simulink library "models"  (Simulink 7.2)
settings: Solver=ode45  SolverMode=SingleTasking  StartTime=0.0  StopTime=10.0  RelTol=1e-3
undefined symbols (not defined in the file or in its folder): actuator_T2_lib, aero, Aero, aero_lib, aftfuel, aftfuel_pos, Am, atmos, b, bias, Bm, Cbar, cg_pos0, cg_shift_gear, constants, DamageModels, Ed_trim_IC, engl_ang, engl_pos, engr_ang, engr_pos, fwdfuel, fwdfuel_pos, GTM_T2, hd_trim_IC, in_tadapton_forced, Inertia0, Inertia_shift_gear, latlonh_IC, MACH_U_nom_IC, Nd_trim_IC, pqr_trim_IC, quat_trim_IC, ref_cg, S, SENSOR, SERVO, symmetric_aero_on, trac_params, use_wind_meas_sim, vehicle_params, w0, xm0
libraries: simulink_need_slupdate x56, models x11, aeroutilslib x6, utility_lib x5, GTM_aerolib x4, model_lib x4, Polyval_lib x3, simulink x2, enginelib x2, engine_T2_lib x1
(part 2 of 4)

== system models/gtm-aero (for V0905)/AuxVars_Reduced ==
  pqr : Inport  OutDataType=sfix(16)  OutScaling=2^0
  aero_env : Inport  Port=2  OutDataType=sfix(16)  OutScaling=2^0
  P : Inport  Port=3  OutDataType=sfix(16)  OutScaling=2^0
  T : Inport  Port=4  OutDataType=sfix(16)  OutScaling=2^0
  Bus Creator : BusCreator  Inputs=6
  Bus Creator1 : BusCreator  Inputs=3
  Bus Selector : BusSelector  OutputSignals=qbar,alpha,beta,vel
  Demux : Demux  Outputs=3
  Gain : Gain  Gain=1/atmos.alt_T0  ParameterDataType=sfix(16)  ParameterScaling=2^0  OutDataType=sfix(16)  OutScaling=2^0
  Gain1 : Gain  Gain=1/atmos.alt_P0  ParameterDataType=sfix(16)  ParameterScaling=2^0  OutDataType=sfix(16)  OutScaling=2^0
  Gain2 : Gain  Gain=180/pi  ParameterDataType=sfix(16)  ParameterScaling=2^0  OutDataType=sfix(16)  OutScaling=2^0
  Gain3 : Gain  Gain=180/pi  ParameterDataType=sfix(16)  ParameterScaling=2^0  OutDataType=sfix(16)  OutScaling=2^0
  Gain5 : Gain  Gain=1/1.689  ParameterDataType=sfix(16)  ParameterScaling=2^0  OutDataType=sfix(16)  OutScaling=2^0
  AuxVars : Outport  OutDataType=sfix(16)  OutScaling=2^0
  State : Outport  Port=2  OutDataType=sfix(16)  OutScaling=2^0
  wires:
  Gain3/1 -> Bus Creator/3  "beta"
  Gain2/1 -> Bus Creator/2  "alpha"
  aero_env/1 -> Bus Selector/1
  P/1 -> Gain1/1
  T/1 -> Gain/1
  Gain1/1 -> Bus Creator/5  "pratio"
  pqr/1 -> Demux/1
  Demux/1 -> Bus Creator1/1  "pb"
  Demux/2 -> Bus Creator1/2  "qb"
  Demux/3 -> Bus Creator1/3  "rb"
  Bus Creator1/1 -> State/1
  Bus Selector/1 -> Bus Creator/1  "<qbar>"
  Bus Selector/2 -> Gain2/1  "<alpha>"
  Bus Selector/3 -> Gain3/1  "<beta>"
  Bus Selector/4 -> Gain5/1  "<vel>"
  Gain/1 -> Bus Creator/6  "tratio"
  Bus Creator/1 -> AuxVars/1
  Gain5/1 -> Bus Creator/4  "tas"

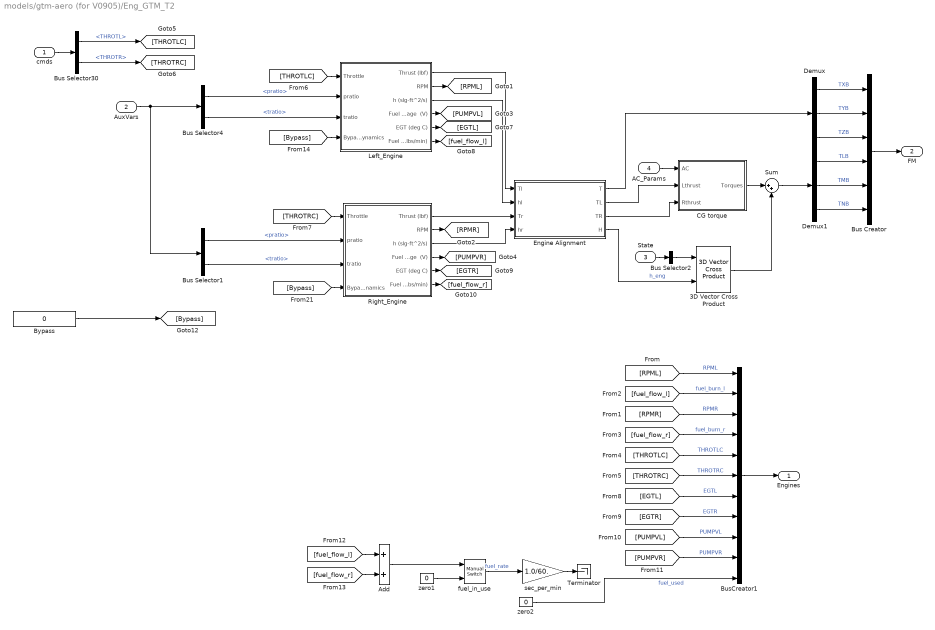
== system models/gtm-aero (for V0905)/Eng_GTM_T2 ==
  cmds : Inport  OutDataType=sfix(16)  OutScaling=2^0
  AuxVars : Inport  Port=2  OutDataType=sfix(16)  OutScaling=2^0
  State : Inport  Port=3  OutDataType=sfix(16)  OutScaling=2^0
  AC_Params : Inport  Port=4  OutDataType=sfix(16)  OutScaling=2^0
  3D Vector Cross Product : aeroutilslib/3D Vector Cross Product  SystemSampleTime=-1
  Add : Sum  OutDataType=sfix(16)  OutScaling=2^-10
  Bus Creator : BusCreator  Inputs=6
  Bus Selector1 : BusSelector  OutputSignals=pratio,tratio
  Bus Selector2 : BusSelector  OutputSignals=pb,qb,rb  OutputAsBus=on
  Bus Selector30 : BusSelector  OutputSignals=THROTL,THROTR
  Bus Selector4 : BusSelector  OutputSignals=pratio,tratio
  BusCreator1 : BusCreator  Inputs=11
  Bypass : Constant  Value=0  OutDataType=sfix(16)  OutScaling=2^0
  CG torque : Subsystem
  Demux : Demux  Outputs=3
  Demux1 : Demux  Outputs=3
  Engine Alignment : Stateflow chart
  Left_Engine : Subsystem  BlockChoice=Jetcat P70b
      settings: AttributesFormatString=%<BlockChoice>  TemplateBlock=enginelib/Engine Model  MemberBlocks=AMT-180,AMT-280,Blank,Jetcat P120SE,Jetcat P70,Jetcat P70b
  Right_Engine : Subsystem  BlockChoice=Jetcat P70b
      settings: AttributesFormatString=%<BlockChoice>  TemplateBlock=enginelib/Engine Model  MemberBlocks=AMT-180,AMT-280,Blank,Jetcat P120SE,Jetcat P70,Jetcat P70b
  Sum : Sum  Inputs=|++  OutDataType=sfix(16)  OutScaling=2^0
  Terminator : Terminator
  fuel_in_use : simulink/Signal Routing/Manual Switch  SystemSampleTime=-1  sw=0  action=0  varsize=off
  sec_per_min : Gain  Gain=1.0/60.  ParameterDataType=sfix(16)  ParameterScaling=2^0  OutDataType=sfix(16)  OutScaling=2^0  SaturateOnIntegerOverflow=on  OutDataTypeStr=Inherit: Same as input  ParamDataTypeStr=Inherit: Same as input
  zero1 : Constant  Value=0  OutDataType=sfix(16)  OutScaling=2^0
  zero2 : Constant  Value=0  OutDataType=sfix(16)  OutScaling=2^0
  Engines : Outport  OutDataType=sfix(16)  OutScaling=2^0
  FM : Outport  Port=2  PortDimensions=6  OutDataType=sfix(16)  OutScaling=2^0
  wires:
  Right_Engine/6(Fuel Flow (lbs/min)) -> [fuel_flow_r]
  Right_Engine/5(EGT (deg C)) -> [EGTR]
  Left_Engine/6(Fuel Flow (lbs/min)) -> [fuel_flow_l]
  Left_Engine/5(EGT (deg C)) -> [EGTL]
  cmds/1 -> Bus Selector30/1
  Demux/2 -> Bus Creator/2  "TYB"
  State/1 -> Bus Selector2/1
  Bus Selector2/1 -> 3D Vector Cross Product/1
  Demux/3 -> Bus Creator/3  "TZB"
  Left_Engine/2(RPM) -> [RPML]
  Left_Engine/4(Fuel Pump Voltage  (V)) -> [PUMPVL]
  Right_Engine/4(Fuel Pump Voltage  (V)) -> [PUMPVR]
  Right_Engine/2(RPM) -> [RPMR]
  Bus Selector1/1 -> Right_Engine/2(pratio)  "<pratio>"
  Bus Selector1/2 -> Right_Engine/3(tratio)  "<tratio>"
  AuxVars/1 -> Bus Selector1/1, Bus Selector4/1
  AC_Params/1 -> CG torque/1(AC)
  Bus Creator/1 -> FM/1
  Bus Selector30/1 -> [THROTLC]  "<THROTL>"
  Bus Selector30/2 -> [THROTRC]  "<THROTR>"
  [THROTLC] -> Left_Engine/1(Throttle)
  [THROTRC] -> Right_Engine/1(Throttle)
  [THROTRC] -> BusCreator1/6  "THROTRC"
  [THROTLC] -> BusCreator1/5  "THROTLC"
  [fuel_flow_r] -> BusCreator1/4  "fuel_burn_r"
  [fuel_flow_l] -> BusCreator1/2  "fuel_burn_l"
  [RPMR] -> BusCreator1/3  "RPMR"
  [RPML] -> BusCreator1/1  "RPML"
  BusCreator1/1 -> Engines/1
  [EGTL] -> BusCreator1/7  "EGTL"
  [EGTR] -> BusCreator1/8  "EGTR"
  [PUMPVL] -> BusCreator1/9  "PUMPVL"
  [PUMPVR] -> BusCreator1/10  "PUMPVR"
  sec_per_min/1 -> Terminator/1
  fuel_in_use/1 -> sec_per_min/1  "fuel_rate"
  zero2/1 -> BusCreator1/11  "fuel_used"
  [fuel_flow_l] -> Add/1
  [fuel_flow_r] -> Add/2
  zero1/1 -> fuel_in_use/2
  Add/1 -> fuel_in_use/1
  Bus Selector4/1 -> Left_Engine/2(pratio)  "<pratio>"
  Bus Selector4/2 -> Left_Engine/3(tratio)  "<tratio>"
  [Bypass] -> Left_Engine/4(BypassDynamics)
  [Bypass] -> Right_Engine/4(BypassDynamics)
  Bypass/1 -> [Bypass]
  Left_Engine/1(Thrust (lbf)) -> Engine Alignment/1(Tl)
  Right_Engine/1(Thrust (lbf)) -> Engine Alignment/3(Tr)
  Demux/1 -> Bus Creator/1  "TXB"
  Left_Engine/3(h (slg-ft^2/s)) -> Engine Alignment/2(hl)
  Right_Engine/3(h (slg-ft^2/s)) -> Engine Alignment/4(hr)
  Engine Alignment/4(H) -> 3D Vector Cross Product/2  "h_eng"
  Engine Alignment/1(T) -> Demux/1
  Engine Alignment/2(TL) -> CG torque/2(Lthrust)
  Engine Alignment/3(TR) -> CG torque/3(Rthrust)
  CG torque/1(Torques) -> Sum/1
  3D Vector Cross Product/1 -> Sum/2
  Sum/1 -> Demux1/1
  Demux1/1 -> Bus Creator/4  "TLB"
  Demux1/2 -> Bus Creator/5  "TMB"
  Demux1/3 -> Bus Creator/6  "TNB"

== system models/gtm-aero (for V0905)/aero surf ganging ==
  u : Inport  OutDataType=sfix(16)  OutScaling=2^0
  Actuator_GTM_T2 (modified) : Subsystem  AncestorBlock=actuator_T2_lib/GTM_T2
  Input Generator (modified) : Subsystem  AncestorBlock=UserContent_lib/Input Generator
  cmds : Outport  OutDataType=sfix(16)  OutScaling=2^0
  wires:
  Input Generator (modified)/2(cmd_stab) -> Actuator_GTM_T2 (modified)/2(cmd_stab)
  Actuator_GTM_T2 (modified)/1(Surface Pos) -> cmds/1
  Input Generator (modified)/1(cmds) -> Actuator_GTM_T2 (modified)/1(cmds)
  u/1 -> Input Generator (modified)/1(Feedback)

== system models/tmp - 1st order sensor model/1st order sensor model ==
  note: VARIABLE RATE LIMIT SERVO MODEL
      | (1st order)
  act_bus : Inport  OutDataType=sfix(16)  OutScaling=2^0
  Bus Selector1 : BusSelector  OutputSignals=effector_limits.u_ulim,effector_limits.u_llim,effector_limits.u_urlim,effector_limits.u_lrlim,u_cmd
  Enforce lower limit : MinMax  Function=max  Inputs=2  OutDataType=sfix(16)  OutScaling=2^-10  OutDataTypeStr=Inherit: Inherit via back propagation  ZeroCross=off
  Enforce lower limit1 : MinMax  Function=max  Inputs=2  OutDataType=sfix(16)  OutScaling=2^-10  OutDataTypeStr=Inherit: Inherit via back propagation  ZeroCross=off
  Enforce upper limit : MinMax  Inputs=2  OutDataType=sfix(16)  OutScaling=2^-10  OutDataTypeStr=Inherit: Inherit via back propagation  ZeroCross=off
  Enforce upper limit1 : MinMax  Inputs=2  OutDataType=sfix(16)  OutScaling=2^-10  OutDataTypeStr=Inherit: Inherit via back propagation  ZeroCross=off
  Sum : Sum  Inputs=|+-  OutDataType=sfix(16)  OutScaling=2^0  SaturateOnIntegerOverflow=on  InputSameDT=on  OutDataTypeStr=Inherit: Same as first input
  Sum1 : Sum  Inputs=|++  OutDataType=sfix(16)  OutScaling=2^0  SaturateOnIntegerOverflow=on  InputSameDT=on  OutDataTypeStr=Inherit: Same as first input
  Sum2 : Sum  Orientation=left  Inputs=-+|  OutDataType=sfix(16)  OutScaling=2^0  SaturateOnIntegerOverflow=on  InputSameDT=on  OutDataTypeStr=Inherit: Same as first input
  W : Gain  Gain=SERVO.w  ParameterDataType=sfix(16)  ParameterScaling=2^0  OutDataType=sfix(16)  OutScaling=2^0  SaturateOnIntegerOverflow=on  OutDataTypeStr=Inherit: Same as input  ParamDataTypeStr=Inherit: Same as input
  anti-windup gain : Gain  Orientation=left  Gain=SERVO.pos_Kaw  ParameterDataType=sfix(16)  ParameterScaling=2^0  OutDataType=sfix(16)  OutScaling=2^0
  pos integrator : Integrator  InitialCondition=SERVO.x0
  u_pos : Outport  OutDataType=sfix(16)  OutScaling=2^0
  wires:
  Enforce upper limit1/1 -> Sum1/1
  Enforce lower limit1/1 -> Enforce upper limit1/2
  W/1 -> Enforce lower limit1/2
  Bus Selector1/3 -> Enforce upper limit1/1  "<u_urlim>"
  Bus Selector1/2 -> Enforce lower limit/1  "<u_llim>"
  Bus Selector1/5 -> Sum/1  "<u_cmd>"
  Sum/1 -> W/1
  Sum1/1 -> pos integrator/1
  anti-windup gain/1 -> Sum1/2
  Sum2/1 -> anti-windup gain/1
  pos integrator/1 -> Enforce lower limit/2, Sum2/1
  Enforce lower limit/1 -> Enforce upper limit/2
  Enforce upper limit/1 -> u_pos/1, Sum/2, Sum2/2
  act_bus/1 -> Bus Selector1/1
  Bus Selector1/1 -> Enforce upper limit/1  "<u_ulim>"
  Bus Selector1/4 -> Enforce lower limit1/1  "<u_lrlim>"

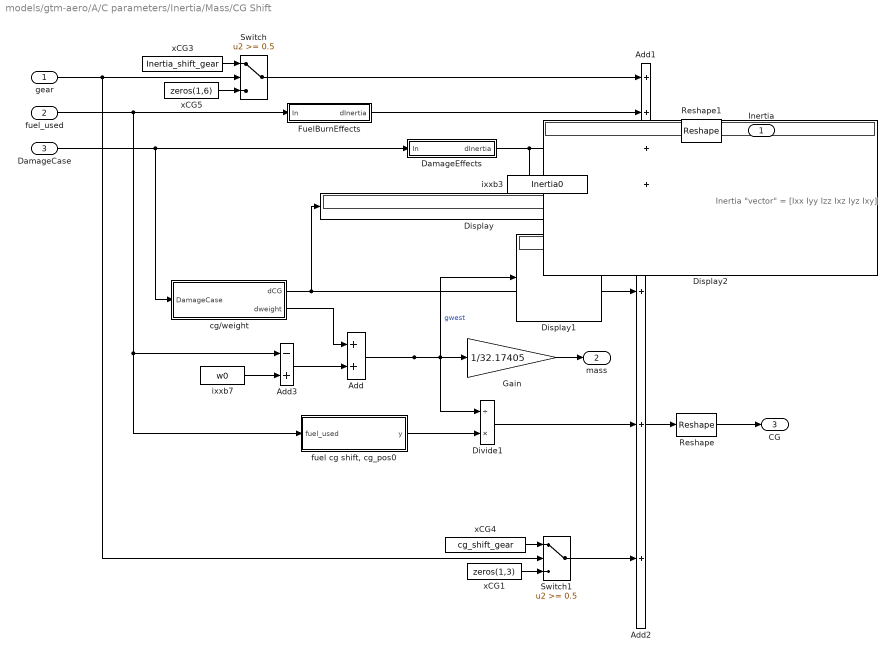
== system models/gtm-aero/A/C parameters/Inertia/Mass/CG Shift ==
  note: Inertia "vector" = [Ixx Iyy Izz Ixz Iyz Ixy]
  gear : Inport  OutDataType=sfix(16)  OutScaling=2^0
  fuel_used : Inport  Port=2  OutDataType=sfix(16)  OutScaling=2^0
  DamageCase : Inport  Port=3  OutDataType=sfix(16)  OutScaling=2^0
  Add : Sum  OutDataType=sfix(16)  OutScaling=2^-10
  Add1 : Sum  Inputs=++++  OutDataType=sfix(16)  OutScaling=2^-10
  Add2 : Sum  Inputs=+++  OutDataType=sfix(16)  OutScaling=2^-10
  Add3 : Sum  Inputs=-+  OutDataType=sfix(16)  OutScaling=2^-10
  DamageEffects : Subsystem
  Display : Display
  Display1 : Display
  Display2 : Display
  Divide1 : Product  Inputs=/*  OutDataType=sfix(16)  OutScaling=2^-10
  FuelBurnEffects : Subsystem
  Gain : Gain  Gain=1/32.17405  ParameterDataType=sfix(16)  ParameterScaling=2^0  OutDataType=sfix(16)  OutScaling=2^0
  Reshape : Reshape
  Reshape1 : Reshape
  Switch : Switch  Threshold=0.5
  Switch1 : Switch  Threshold=0.5
  cg/weight : Subsystem
  "fuel cg shift, cg_pos0" : Stateflow chart
  ixxb3 : Constant  Value=Inertia0  OutDataType=sfix(16)  OutScaling=2^0
  ixxb7 : Constant  Value=w0  OutDataType=sfix(16)  OutScaling=2^0
  xCG1 : Constant  Value=zeros(1,3)  OutDataType=sfix(16)  OutScaling=2^0
  xCG3 : Constant  Value=Inertia_shift_gear  OutDataType=sfix(16)  OutScaling=2^0
  xCG4 : Constant  Value=cg_shift_gear  OutDataType=sfix(16)  OutScaling=2^0
  xCG5 : Constant  Value=zeros(1,6)  OutDataType=sfix(16)  OutScaling=2^0
  Inertia : Outport  OutDataType=sfix(16)  OutScaling=2^0
  mass : Outport  Port=2  OutDataType=sfix(16)  OutScaling=2^0
  CG : Outport  Port=3  OutDataType=sfix(16)  OutScaling=2^0
  wires:
  "fuel cg shift, cg_pos0"/1(y) -> Divide1/2
  Divide1/1 -> Add2/2
  Reshape1/1 -> Inertia/1
  Reshape/1 -> CG/1
  cg/weight/2(dweight) -> Add/1
  gear/1 -> Switch1/2, Switch/2
  cg/weight/1(dCG) -> Display/1, Add2/1
  Add3/1 -> Add/2
  xCG1/1 -> Switch1/3
  xCG4/1 -> Switch1/1
  Switch1/1 -> Add2/3
  ixxb7/1 -> Add3/2
  Gain/1 -> mass/1
  Add2/1 -> Reshape/1
  Add/1 -> Display1/1, Divide1/1, Gain/1  "gwest"
  DamageCase/1 -> cg/weight/1(DamageCase), DamageEffects/1(In)
  DamageEffects/1(dInertia) -> Display2/1, Add1/3
  ixxb3/1 -> Add1/4
  fuel_used/1 -> "fuel cg shift, cg_pos0"/1(fuel_used), Add3/1, FuelBurnEffects/1(In)
  xCG5/1 -> Switch/3
  xCG3/1 -> Switch/1
  Add1/1 -> Reshape1/1
  Switch/1 -> Add1/1
  FuelBurnEffects/1(dInertia) -> Add1/2

== system models/gtm-aero/A/C parameters/TriggerDamage ==
  From Workspace : FromWorkspace  VariableName=[0 0; DamageOnsetTime DamageCase]  Interpolate=off  OutputAfterFinalValue=Holding final value
  damagecase : Outport  OutDataType=sfix(16)  OutScaling=2^0
  wires:
  From Workspace/1 -> damagecase/1

== system models/gtm-aero/Aero_GTM_T2/Coefficent Evaluation ==
  C6 Body : Inport  OutDataType=sfix(16)  OutScaling=2^0
  qbar : Inport  Port=2  OutDataType=sfix(16)  OutScaling=2^0
  Cg : Inport  Port=3  OutDataType=sfix(16)  OutScaling=2^0
  Cp : Inport  Port=4  OutDataType=sfix(16)  OutScaling=2^0
  3D Vector Cross Product : Subsystem  AncestorBlock=aeroutilslib/3D Vector Cross Product
  Demux : Demux  Outputs=[3 3]
  Gain2 : Gain  Gain=Sref  ParameterDataType=sfix(16)  ParameterScaling=2^0  OutDataType=sfix(16)  OutScaling=2^0  SaturateOnIntegerOverflow=on  OutDataTypeStr=Inherit: Same as input  ParamDataTypeStr=Inherit: Same as input
  Product : Product  OutDataType=sfix(16)  OutScaling=2^0  SaturateOnIntegerOverflow=on  InputSameDT=on  OutDataTypeStr=Inherit: Same as first input
  Reference Lengths : Gain  Gain=[b cbar b]  ParameterDataType=sfix(16)  ParameterScaling=2^0  OutDataType=sfix(16)  OutScaling=2^0  SaturateOnIntegerOverflow=on  OutDataTypeStr=Inherit: Same as input  ParamDataTypeStr=Inherit: Same as input
  Sum : Sum  Inputs=-+  OutDataType=sfix(16)  OutScaling=2^0  SaturateOnIntegerOverflow=on
  Sum1 : Sum  Inputs=++|  OutDataType=sfix(16)  OutScaling=2^0  SaturateOnIntegerOverflow=on
  Forces : Outport  OutDataType=sfix(16)  OutScaling=2^0
  Moments : Outport  Port=2  OutDataType=sfix(16)  OutScaling=2^0
  wires:
  Sum/1 -> 3D Vector Cross Product/1(A)
  Cg/1 -> Sum/1
  Cp/1 -> Sum/2
  C6 Body/1 -> Product/1
  qbar/1 -> Product/2
  Product/1 -> Gain2/1
  Gain2/1 -> Demux/1
  Demux/2 -> Reference Lengths/1
  Demux/1 -> 3D Vector Cross Product/2(B), Forces/1
  Reference Lengths/1 -> Sum1/2
  Sum1/1 -> Moments/1
  3D Vector Cross Product/1(AxB) -> Sum1/1

== system models/gtm-aero/Aero_GTM_T2/Dynamic Derviatives ==
  alpha : Inport  OutDataType=sfix(16)  OutScaling=2^0
  beta : Inport  Port=2  OutDataType=sfix(16)  OutScaling=2^0
  TAS : Inport  Port=3  OutDataType=sfix(16)  OutScaling=2^0
  pqr : Inport  Port=4  OutDataType=sfix(16)  OutScaling=2^0
  AC_Params : Inport  Port=5  OutDataType=sfix(16)  OutScaling=2^0
  AC_Params1 : InportShadow  Port=5  OutDataType=sfix(16)  OutScaling=2^0  LatchByCopyingInsideSignal=off
  AC_Params_Dup1 : InportShadow  Port=5  OutDataType=sfix(16)  OutScaling=2^0  LatchByCopyingInsideSignal=off
  Bus Selector : BusSelector  OutputSignals=DamageCase
  Data Type Conversion : DataTypeConversion  OutDataTypeMode=uint32  OutDataType=sfix(16)  OutScaling=2^0  OutDataTypeStr=uint32  RndMeth=Nearest
  Forced Oscillation with Damage Increments : Subsystem
  Merge : Merge  InitialOutput=zeros(6,1)
  Rotary Blended  UnDamaged Case : Subsystem
  Switch Case : SwitchCase  CaseConditions={[1,2,3,4,5,6]}
  TAS1 : InportShadow  Port=3  OutDataType=sfix(16)  OutScaling=2^0  LatchByCopyingInsideSignal=off
  alpha_Dup1 : InportShadow  Port=1  OutDataType=sfix(16)  OutScaling=2^0  LatchByCopyingInsideSignal=off
  pqr_Dup1 : InportShadow  Port=4  OutDataType=sfix(16)  OutScaling=2^0  LatchByCopyingInsideSignal=off
  dC6 : Outport  OutDataType=sfix(16)  OutScaling=2^0
  wires:
  Forced Oscillation with Damage Increments/1(dC6) -> Merge/1
  [ndx] -> Forced Oscillation with Damage Increments/5(DamageCase)
  AC_Params1/1 -> Forced Oscillation with Damage Increments/4(AC_Params)
  pqr_Dup1/1 -> Forced Oscillation with Damage Increments/3(pqr)
  TAS1/1 -> Forced Oscillation with Damage Increments/2(TAS)
  alpha_Dup1/1 -> Forced Oscillation with Damage Increments/1(alpha)
  [ndx] -> Switch Case/1
  Data Type Conversion/1 -> [ndx]
  AC_Params_Dup1/1 -> Bus Selector/1
  Bus Selector/1 -> Data Type Conversion/1  "<DamageCase>"
  Rotary Blended  UnDamaged Case/1(dC6) -> Merge/2
  Switch Case/2 -> Rotary Blended  UnDamaged Case/Action
  Switch Case/1 -> Forced Oscillation with Damage Increments/Action
  Merge/1 -> dC6/1
  AC_Params/1 -> Rotary Blended  UnDamaged Case/5(AC_Params)
  pqr/1 -> Rotary Blended  UnDamaged Case/4(pqr)
  TAS/1 -> Rotary Blended  UnDamaged Case/3(TAS)
  beta/1 -> Rotary Blended  UnDamaged Case/2(beta)
  alpha/1 -> Rotary Blended  UnDamaged Case/1(alpha)

== system models/gtm-aero/Aero_GTM_T2/Label ==
  If : Inport  OutDataType=sfix(16)  OutScaling=2^0
  Im : Inport  Port=2  OutDataType=sfix(16)  OutScaling=2^0
  Bus Creator1 : BusCreator  Inputs=6
  Demux1 : Demux  Outputs=3
  Demux3 : Demux  Outputs=3
  O : Outport  OutDataType=sfix(16)  OutScaling=2^0
  wires:
  Bus Creator1/1 -> O/1
  If/1 -> Demux1/1
  Demux1/1 -> Bus Creator1/1  "XB"
  Demux1/2 -> Bus Creator1/2  "YB"
  Demux1/3 -> Bus Creator1/3  "ZB"
  Demux3/1 -> Bus Creator1/4  "LB"
  Demux3/2 -> Bus Creator1/5  "MB"
  Demux3/3 -> Bus Creator1/6  "NB"
  Im/1 -> Demux3/1

== system models/gtm-aero/aero surf ganging/Actuator_GTM_T2 (modified) ==
  cmds : Inport  OutDataType=sfix(16)  OutScaling=2^0
  cmd_stab : Inport  Port=2  OutDataType=sfix(16)  OutScaling=2^0
  Brake : Saturate  UpperLimit=1.0  LowerLimit=0.0
  Bus Selector2 : BusSelector  OutputSignals=ELLOBC,ELLIBC,ELROBC,ELRIBC,AILLC,AILRC,RUDUPC,RUDLOC,SPLLIBC,SPLLOBC,SPLRIBC,SPLROBC,FLAPLIC,FLAPLOC,FLAPRIC,FLAPROC,GEARC,BRAKEC,THROTLC,THROTRC,STEERC
  Gear : Saturate  UpperLimit=1.0  LowerLimit=0.0
  Gear1 : Constant  Value=bias.stabilizer*0  OutDataType=sfix(16)  OutScaling=2^0
  Ground : Ground
  Label : Subsystem
  Mux : Mux  Inputs=22
  Sum : Sum  Inputs=++|  OutDataType=sfix(16)  OutScaling=2^0
  Sum3 : Sum  Inputs=|++  OutDataType=sfix(16)  OutScaling=2^0
  Surface Allocation : Subsystem
  Surface Pos : Outport  OutDataType=sfix(16)  OutScaling=2^0
  wires:
  Sum/1 -> Label/1(I)
  Label/1(O) -> Surface Pos/1
  Ground/1 -> Surface Allocation/1(I)
  Bus Selector2/13 -> Mux/13  "<FLAPLIC>"
  Bus Selector2/14 -> Mux/14  "<FLAPLOC>"
  Bus Selector2/15 -> Mux/15  "<FLAPRIC>"
  Bus Selector2/16 -> Mux/16  "<FLAPROC>"
  Bus Selector2/17 -> Gear/1  "<GEARC>"
  Bus Selector2/18 -> Brake/1  "<BRAKEC>"
  Mux/1 -> Sum/2
  Bus Selector2/1 -> Mux/1  "<ELLOBC>"
  Bus Selector2/2 -> Mux/2  "<ELLIBC>"
  Bus Selector2/3 -> Mux/3  "<ELROBC>"
  Bus Selector2/4 -> Mux/4  "<ELRIBC>"
  Bus Selector2/5 -> Mux/5  "<AILLC>"
  Bus Selector2/6 -> Mux/6  "<AILRC>"
  Bus Selector2/7 -> Mux/7  "<RUDUPC>"
  Bus Selector2/8 -> Mux/8  "<RUDLOC>"
  Bus Selector2/9 -> Mux/9  "<SPLLIBC>"
  Bus Selector2/10 -> Mux/10  "<SPLLOBC>"
  Bus Selector2/11 -> Mux/11  "<SPLRIBC>"
  Bus Selector2/12 -> Mux/12  "<SPLROBC>"
  Gear/1 -> Mux/18
  Brake/1 -> Mux/19
  cmds/1 -> Bus Selector2/1
  Surface Allocation/1(O) -> Sum/1
  Bus Selector2/19 -> Mux/20  "<THROTLC>"
  Bus Selector2/20 -> Mux/21  "<THROTRC>"
  Bus Selector2/21 -> Mux/22  "<STEERC>"
  cmd_stab/1 -> Sum3/1
  Gear1/1 -> Sum3/2
  Sum3/1 -> Mux/17

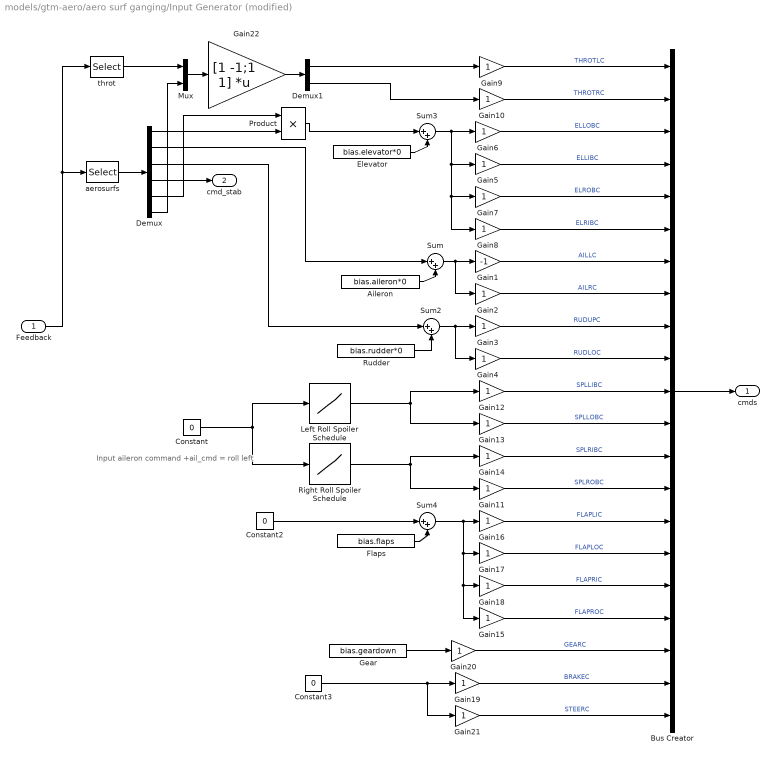
== system models/gtm-aero/aero surf ganging/Input Generator (modified) ==
  note: Input aileron command
      | +ail_cmd = roll left
  Feedback : Inport  OutDataType=sfix(16)  OutScaling=2^0
  Aileron : Constant  Value=bias.aileron*0  OutDataType=sfix(16)  OutScaling=2^0
  Bus Creator : BusCreator  Inputs=21
  Constant : Constant  Value=0  OutDataType=sfix(16)  OutScaling=2^0
  Constant2 : Constant  Value=0  OutDataType=sfix(16)  OutScaling=2^0
  Constant3 : Constant  Value=0  OutDataType=sfix(16)  OutScaling=2^0
  Demux : Demux  Outputs=6
  Demux1 : Demux  Outputs=2
  Elevator : Constant  Value=bias.elevator*0  OutDataType=sfix(16)  OutScaling=2^0
  Flaps : Constant  Value=bias.flaps  OutDataType=sfix(16)  OutScaling=2^0
  Gain1 : Gain  Gain=-1  ParameterDataType=sfix(16)  ParameterScaling=2^0  OutDataType=sfix(16)  OutScaling=2^0  SaturateOnIntegerOverflow=on  OutDataTypeStr=Inherit: Same as input  ParamDataTypeStr=Inherit: Same as input
  Gain{2..21} (20 alike) : Gain  ParameterDataType=sfix(16)  ParameterScaling=2^0  OutDataType=sfix(16)  OutScaling=2^0  SaturateOnIntegerOverflow=on  OutDataTypeStr=Inherit: Same as input  ParamDataTypeStr=Inherit: Same as input
  Gain22 : Gain  Gain=[1 -1;1 1]  Multiplication=Matrix(K*u)  ParameterDataType=sfix(16)  ParameterScaling=2^0  OutDataType=sfix(16)  OutScaling=2^0  SaturateOnIntegerOverflow=on  OutDataTypeStr=Inherit: Same as input  ParamDataTypeStr=Inherit: Same as input
  Gear : Constant  Value=bias.geardown  OutDataType=sfix(16)  OutScaling=2^0
  Left Roll Spoiler Schedule : Lookup  InputValues="[-20\t-11.76\t-2.36\t0\t2.36\t11.76\t20\t]"  Table=[0 0 0 0 0 9 45]  LookUpMeth=Interpolation-Use End Values  OutDataType=sfix(16)  OutScaling=2^0
  Mux : Mux  Inputs=2
  Product : Product  OutDataType=sfix(16)  OutScaling=2^0  RndMeth=Zero
  Right Roll Spoiler Schedule : Lookup  InputValues="[-20\t-11.76\t-2.36\t0\t2.36\t11.76\t20\t]"  Table=[45 9 0 0 0 0 0]  LookUpMeth=Interpolation-Use End Values  OutDataType=sfix(16)  OutScaling=2^0
  Rudder : Constant  Value=bias.rudder*0  OutDataType=sfix(16)  OutScaling=2^0
  Sum{,2..4} (4 alike) : Sum  Inputs=|++  OutDataType=sfix(16)  OutScaling=2^0
  aerosurfs : Selector  InputPortWidth=num_u  IndexOptions=Index vector (dialog)  Indices=vane_idx  OutputSizes=1
  throt : Selector  InputPortWidth=num_u  IndexOptions=Index vector (dialog)  Indices=throttle_idx  OutputSizes=1
  cmds : Outport  OutDataType=sfix(16)  OutScaling=2^0
  cmd_stab : Outport  Port=2  OutDataType=sfix(16)  OutScaling=2^0
  wires:
  Constant/1 -> Right Roll Spoiler Schedule/1, Left Roll Spoiler Schedule/1
  Right Roll Spoiler Schedule/1 -> Gain11/1, Gain14/1
  Left Roll Spoiler Schedule/1 -> Gain13/1, Gain12/1
  Gain12/1 -> Bus Creator/11  "SPLLIBC"
  Gain13/1 -> Bus Creator/12  "SPLLOBC"
  Gain14/1 -> Bus Creator/13  "SPLRIBC"
  Gain11/1 -> Bus Creator/14  "SPLROBC"
  Gain16/1 -> Bus Creator/15  "FLAPLIC"
  Gain17/1 -> Bus Creator/16  "FLAPLOC"
  Gain18/1 -> Bus Creator/17  "FLAPRIC"
  Gain15/1 -> Bus Creator/18  "FLAPROC"
  Gain9/1 -> Bus Creator/1  "THROTLC"
  Gain10/1 -> Bus Creator/2  "THROTRC"
  Gain5/1 -> Bus Creator/4  "ELLIBC"
  Gain6/1 -> Bus Creator/3  "ELLOBC"
  Gain7/1 -> Bus Creator/5  "ELROBC"
  Gain8/1 -> Bus Creator/6  "ELRIBC"
  Gain1/1 -> Bus Creator/7  "AILLC"
  Gain2/1 -> Bus Creator/8  "AILRC"
  Gain3/1 -> Bus Creator/9  "RUDUPC"
  Gain4/1 -> Bus Creator/10  "RUDLOC"
  Sum3/1 -> Gain6/1, Gain5/1, Gain7/1, Gain8/1
  Aileron/1 -> Sum/2
  Elevator/1 -> Sum3/2
  Sum/1 -> Gain1/1, Gain2/1
  Sum2/1 -> Gain3/1, Gain4/1
  Rudder/1 -> Sum2/2
  Flaps/1 -> Sum4/2
  Constant2/1 -> Sum4/1
  Sum4/1 -> Gain16/1, Gain17/1, Gain18/1, Gain15/1
  Demux/2 -> Sum/1
  Demux/3 -> Sum2/1
  Gain19/1 -> Bus Creator/20  "BRAKEC"
  Gear/1 -> Gain20/1
  Constant3/1 -> Gain19/1, Gain21/1
  Bus Creator/1 -> cmds/1
  Feedback/1 -> throt/1, aerosurfs/1
  Gain20/1 -> Bus Creator/19  "GEARC"
  Gain21/1 -> Bus Creator/21  "STEERC"
  aerosurfs/1 -> Demux/1
  Demux/4 -> cmd_stab/1
  Product/1 -> Sum3/1
  Demux/1 -> Product/2
  Demux/5 -> Product/1
  Demux/6 -> Mux/2
  throt/1 -> Mux/1
  Mux/1 -> Gain22/1
  Gain22/1 -> Demux1/1
  Demux1/1 -> Gain9/1
  Demux1/2 -> Gain10/1

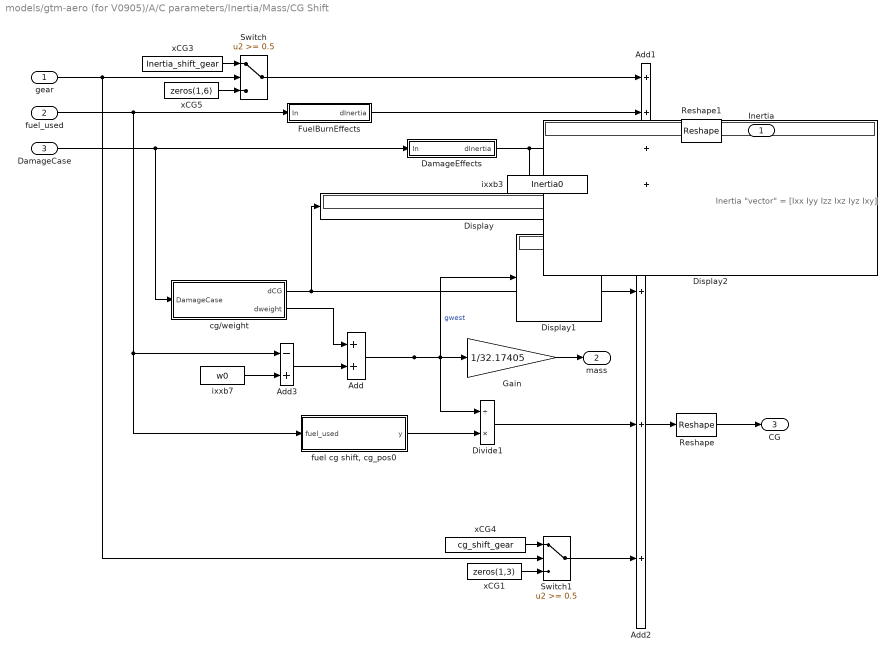
== system models/gtm-aero (for V0905)/A/C parameters/Inertia/Mass/CG Shift ==
  note: Inertia "vector" = [Ixx Iyy Izz Ixz Iyz Ixy]
  gear : Inport  OutDataType=sfix(16)  OutScaling=2^0
  fuel_used : Inport  Port=2  OutDataType=sfix(16)  OutScaling=2^0
  DamageCase : Inport  Port=3  OutDataType=sfix(16)  OutScaling=2^0
  Add : Sum  OutDataType=sfix(16)  OutScaling=2^-10
  Add1 : Sum  Inputs=++++  OutDataType=sfix(16)  OutScaling=2^-10
  Add2 : Sum  Inputs=+++  OutDataType=sfix(16)  OutScaling=2^-10
  Add3 : Sum  Inputs=-+  OutDataType=sfix(16)  OutScaling=2^-10
  DamageEffects : Subsystem
  Display : Display
  Display1 : Display
  Display2 : Display
  Divide1 : Product  Inputs=/*  OutDataType=sfix(16)  OutScaling=2^-10
  FuelBurnEffects : Subsystem
  Gain : Gain  Gain=1/32.17405  ParameterDataType=sfix(16)  ParameterScaling=2^0  OutDataType=sfix(16)  OutScaling=2^0
  Reshape : Reshape
  Reshape1 : Reshape
  Switch : Switch  Threshold=0.5
  Switch1 : Switch  Threshold=0.5
  cg/weight : Subsystem
  "fuel cg shift, cg_pos0" : Stateflow chart
  ixxb3 : Constant  Value=Inertia0  OutDataType=sfix(16)  OutScaling=2^0
  ixxb7 : Constant  Value=w0  OutDataType=sfix(16)  OutScaling=2^0
  xCG1 : Constant  Value=zeros(1,3)  OutDataType=sfix(16)  OutScaling=2^0
  xCG3 : Constant  Value=Inertia_shift_gear  OutDataType=sfix(16)  OutScaling=2^0
  xCG4 : Constant  Value=cg_shift_gear  OutDataType=sfix(16)  OutScaling=2^0
  xCG5 : Constant  Value=zeros(1,6)  OutDataType=sfix(16)  OutScaling=2^0
  Inertia : Outport  OutDataType=sfix(16)  OutScaling=2^0
  mass : Outport  Port=2  OutDataType=sfix(16)  OutScaling=2^0
  CG : Outport  Port=3  OutDataType=sfix(16)  OutScaling=2^0
  wires:
  FuelBurnEffects/1(dInertia) -> Add1/2
  Switch/1 -> Add1/1
  Add1/1 -> Reshape1/1
  xCG3/1 -> Switch/1
  xCG5/1 -> Switch/3
  fuel_used/1 -> FuelBurnEffects/1(In), Add3/1, "fuel cg shift, cg_pos0"/1(fuel_used)
  ixxb3/1 -> Add1/4
  DamageEffects/1(dInertia) -> Add1/3, Display2/1
  DamageCase/1 -> DamageEffects/1(In), cg/weight/1(DamageCase)
  Add/1 -> Gain/1, Divide1/1, Display1/1  "gwest"
  Add2/1 -> Reshape/1
  Gain/1 -> mass/1
  ixxb7/1 -> Add3/2
  Switch1/1 -> Add2/3
  xCG4/1 -> Switch1/1
  xCG1/1 -> Switch1/3
  Add3/1 -> Add/2
  cg/weight/1(dCG) -> Add2/1, Display/1
  gear/1 -> Switch/2, Switch1/2
  cg/weight/2(dweight) -> Add/1
  Reshape/1 -> CG/1
  Reshape1/1 -> Inertia/1
  Divide1/1 -> Add2/2
  "fuel cg shift, cg_pos0"/1(y) -> Divide1/2

== system models/gtm-aero (for V0905)/A/C parameters/TriggerDamage ==
  From Workspace : FromWorkspace  VariableName=[0 0; DamageOnsetTime DamageCase]  Interpolate=off  OutputAfterFinalValue=Holding final value
  damagecase : Outport  OutDataType=sfix(16)  OutScaling=2^0
  wires:
  From Workspace/1 -> damagecase/1

== system models/gtm-aero (for V0905)/Aero_GTM_T2/Coefficent Evaluation ==
  C6 Body : Inport  OutDataType=sfix(16)  OutScaling=2^0
  qbar : Inport  Port=2  OutDataType=sfix(16)  OutScaling=2^0
  Cg : Inport  Port=3  OutDataType=sfix(16)  OutScaling=2^0
  Cp : Inport  Port=4  OutDataType=sfix(16)  OutScaling=2^0
  3D Vector Cross Product : Subsystem  AncestorBlock=aeroutilslib/3D Vector Cross Product
  Demux : Demux  Outputs=[3 3]
  Gain2 : Gain  Gain=Sref  ParameterDataType=sfix(16)  ParameterScaling=2^0  OutDataType=sfix(16)  OutScaling=2^0  SaturateOnIntegerOverflow=on  OutDataTypeStr=Inherit: Same as input  ParamDataTypeStr=Inherit: Same as input
  Product : Product  OutDataType=sfix(16)  OutScaling=2^0  SaturateOnIntegerOverflow=on  InputSameDT=on  OutDataTypeStr=Inherit: Same as first input
  Reference Lengths : Gain  Gain=[b cbar b]  ParameterDataType=sfix(16)  ParameterScaling=2^0  OutDataType=sfix(16)  OutScaling=2^0  SaturateOnIntegerOverflow=on  OutDataTypeStr=Inherit: Same as input  ParamDataTypeStr=Inherit: Same as input
  Sum : Sum  Inputs=-+  OutDataType=sfix(16)  OutScaling=2^0  SaturateOnIntegerOverflow=on
  Sum1 : Sum  Inputs=++|  OutDataType=sfix(16)  OutScaling=2^0  SaturateOnIntegerOverflow=on
  Forces : Outport  OutDataType=sfix(16)  OutScaling=2^0
  Moments : Outport  Port=2  OutDataType=sfix(16)  OutScaling=2^0
  wires:
  3D Vector Cross Product/1(AxB) -> Sum1/1
  Sum1/1 -> Moments/1
  Reference Lengths/1 -> Sum1/2
  Demux/1 -> Forces/1, 3D Vector Cross Product/2(B)
  Demux/2 -> Reference Lengths/1
  Gain2/1 -> Demux/1
  Product/1 -> Gain2/1
  qbar/1 -> Product/2
  C6 Body/1 -> Product/1
  Cp/1 -> Sum/2
  Cg/1 -> Sum/1
  Sum/1 -> 3D Vector Cross Product/1(A)

== system models/gtm-aero (for V0905)/Aero_GTM_T2/Dynamic Derviatives ==
  alpha : Inport  OutDataType=sfix(16)  OutScaling=2^0
  beta : Inport  Port=2  OutDataType=sfix(16)  OutScaling=2^0
  TAS : Inport  Port=3  OutDataType=sfix(16)  OutScaling=2^0
  pqr : Inport  Port=4  OutDataType=sfix(16)  OutScaling=2^0
  AC_Params : Inport  Port=5  OutDataType=sfix(16)  OutScaling=2^0
  AC_Params1 : InportShadow  Port=5  OutDataType=sfix(16)  OutScaling=2^0  LatchByCopyingInsideSignal=off
  AC_Params_Dup1 : InportShadow  Port=5  OutDataType=sfix(16)  OutScaling=2^0  LatchByCopyingInsideSignal=off
  Bus Selector : BusSelector  OutputSignals=DamageCase
  Data Type Conversion : DataTypeConversion  OutDataTypeMode=uint32  OutDataType=sfix(16)  OutScaling=2^0  OutDataTypeStr=uint32  RndMeth=Nearest
  Forced Oscillation with Damage Increments : Subsystem
  Merge : Merge  InitialOutput=zeros(6,1)
  Rotary Blended  UnDamaged Case : Subsystem
  Switch Case : SwitchCase  CaseConditions={[1,2,3,4,5,6]}
  TAS1 : InportShadow  Port=3  OutDataType=sfix(16)  OutScaling=2^0  LatchByCopyingInsideSignal=off
  alpha_Dup1 : InportShadow  Port=1  OutDataType=sfix(16)  OutScaling=2^0  LatchByCopyingInsideSignal=off
  pqr_Dup1 : InportShadow  Port=4  OutDataType=sfix(16)  OutScaling=2^0  LatchByCopyingInsideSignal=off
  dC6 : Outport  OutDataType=sfix(16)  OutScaling=2^0
  wires:
  alpha/1 -> Rotary Blended  UnDamaged Case/1(alpha)
  beta/1 -> Rotary Blended  UnDamaged Case/2(beta)
  TAS/1 -> Rotary Blended  UnDamaged Case/3(TAS)
  pqr/1 -> Rotary Blended  UnDamaged Case/4(pqr)
  AC_Params/1 -> Rotary Blended  UnDamaged Case/5(AC_Params)
  Merge/1 -> dC6/1
  Switch Case/1 -> Forced Oscillation with Damage Increments/Action
  Switch Case/2 -> Rotary Blended  UnDamaged Case/Action
  Rotary Blended  UnDamaged Case/1(dC6) -> Merge/2
  Bus Selector/1 -> Data Type Conversion/1  "<DamageCase>"
  AC_Params_Dup1/1 -> Bus Selector/1
  Data Type Conversion/1 -> [ndx]
  [ndx] -> Switch Case/1
  alpha_Dup1/1 -> Forced Oscillation with Damage Increments/1(alpha)
  TAS1/1 -> Forced Oscillation with Damage Increments/2(TAS)
  pqr_Dup1/1 -> Forced Oscillation with Damage Increments/3(pqr)
  AC_Params1/1 -> Forced Oscillation with Damage Increments/4(AC_Params)
  [ndx] -> Forced Oscillation with Damage Increments/5(DamageCase)
  Forced Oscillation with Damage Increments/1(dC6) -> Merge/1

== system models/gtm-aero (for V0905)/Aero_GTM_T2/Label ==
  If : Inport  OutDataType=sfix(16)  OutScaling=2^0
  Im : Inport  Port=2  OutDataType=sfix(16)  OutScaling=2^0
  Bus Creator1 : BusCreator  Inputs=6
  Demux1 : Demux  Outputs=3
  Demux3 : Demux  Outputs=3
  O : Outport  OutDataType=sfix(16)  OutScaling=2^0
  wires:
  Im/1 -> Demux3/1
  Demux3/3 -> Bus Creator1/6  "NB"
  Demux3/2 -> Bus Creator1/5  "MB"
  Demux3/1 -> Bus Creator1/4  "LB"
  Demux1/3 -> Bus Creator1/3  "ZB"
  Demux1/2 -> Bus Creator1/2  "YB"
  Demux1/1 -> Bus Creator1/1  "XB"
  If/1 -> Demux1/1
  Bus Creator1/1 -> O/1

== system models/gtm-aero (for V0905)/Eng_GTM_T2/CG torque ==
  AC : Inport  OutDataType=sfix(16)  OutScaling=2^0
  Lthrust : Inport  Port=2  OutDataType=sfix(16)  OutScaling=2^0
  Rthrust : Inport  Port=3  OutDataType=sfix(16)  OutScaling=2^0
  3D Vector Cross Product : aeroutilslib/3D Vector Cross Product  SystemSampleTime=-1
  3D Vector Cross Product1 : aeroutilslib/3D Vector Cross Product  SystemSampleTime=-1
  Bus Selector30 : BusSelector  OutputSignals=LfEng,CG,RtEng
  Sum1 : Sum  OutDataType=sfix(16)  OutScaling=2^0  SaturateOnIntegerOverflow=on  InputSameDT=on  OutDataTypeStr=Inherit: Same as first input
  Sum6 : Sum  Inputs=+-  OutDataType=sfix(16)  OutScaling=2^0  SaturateOnIntegerOverflow=on  InputSameDT=on  OutDataTypeStr=Inherit: Same as first input
  Sum7 : Sum  Inputs=-+  OutDataType=sfix(16)  OutScaling=2^0  SaturateOnIntegerOverflow=on  InputSameDT=on  OutDataTypeStr=Inherit: Same as first input
  Torques : Outport  OutDataType=sfix(16)  OutScaling=2^0
  wires:
  AC/1 -> Bus Selector30/1
  Bus Selector30/2 -> Sum7/1, Sum6/2  "<CG>"
  Lthrust/1 -> 3D Vector Cross Product1/2
  Rthrust/1 -> 3D Vector Cross Product/2
  Sum7/1 -> 3D Vector Cross Product/1
  Sum6/1 -> 3D Vector Cross Product1/1
  3D Vector Cross Product1/1 -> Sum1/1
  3D Vector Cross Product/1 -> Sum1/2
  Sum1/1 -> Torques/1
  Bus Selector30/3 -> Sum7/2  "<RtEng>"
  Bus Selector30/1 -> Sum6/1  "<LfEng>"

== system models/gtm-aero (for V0905)/Eng_GTM_T2/Left_Engine ==
  Throttle : Inport  OutDataType=sfix(16)  OutScaling=2^0
  pratio : Inport  Port=2  OutDataType=sfix(16)  OutScaling=2^0
  tratio : Inport  Port=3  OutDataType=sfix(16)  OutScaling=2^0
  BypassDynamics : Inport  Port=4  OutDataType=sfix(16)  OutScaling=2^0
  Jetcat P70b : enginelib/Jetcat P70b  SystemSampleTime=-1
  term4 : Terminator
  Thrust (lbf) : Outport  OutDataType=sfix(16)  OutScaling=2^0
  RPM : Outport  Port=2  OutDataType=sfix(16)  OutScaling=2^0
  h (slg-ft^2/s) : Outport  Port=3  OutDataType=sfix(16)  OutScaling=2^0
  Fuel Pump Voltage  (V) : Outport  Port=4  OutDataType=sfix(16)  OutScaling=2^0
  EGT (deg C) : Outport  Port=5  OutDataType=sfix(16)  OutScaling=2^0
  Fuel Flow (lbs/min) : Outport  Port=6  OutDataType=sfix(16)  OutScaling=2^0
  wires:
  BypassDynamics/1 -> term4/1
  Jetcat P70b/6 -> EGT (deg C)/1
  Jetcat P70b/5 -> Fuel Pump Voltage  (V)/1
  Jetcat P70b/4 -> Fuel Flow (lbs/min)/1
  Jetcat P70b/3 -> h (slg-ft^2/s)/1
  Jetcat P70b/2 -> RPM/1
  Jetcat P70b/1 -> Thrust (lbf)/1
  tratio/1 -> Jetcat P70b/3
  pratio/1 -> Jetcat P70b/2
  Throttle/1 -> Jetcat P70b/1

== system models/gtm-aero (for V0905)/Eng_GTM_T2/Right_Engine ==
  Throttle : Inport  OutDataType=sfix(16)  OutScaling=2^0
  pratio : Inport  Port=2  OutDataType=sfix(16)  OutScaling=2^0
  tratio : Inport  Port=3  OutDataType=sfix(16)  OutScaling=2^0
  BypassDynamics : Inport  Port=4  OutDataType=sfix(16)  OutScaling=2^0
  Jetcat P70b : enginelib/Jetcat P70b  SystemSampleTime=-1
  term4 : Terminator
  Thrust (lbf) : Outport  OutDataType=sfix(16)  OutScaling=2^0
  RPM : Outport  Port=2  OutDataType=sfix(16)  OutScaling=2^0
  h (slg-ft^2/s) : Outport  Port=3  OutDataType=sfix(16)  OutScaling=2^0
  Fuel Pump Voltage  (V) : Outport  Port=4  OutDataType=sfix(16)  OutScaling=2^0
  EGT (deg C) : Outport  Port=5  OutDataType=sfix(16)  OutScaling=2^0
  Fuel Flow (lbs/min) : Outport  Port=6  OutDataType=sfix(16)  OutScaling=2^0
  wires:
  BypassDynamics/1 -> term4/1
  Jetcat P70b/6 -> EGT (deg C)/1
  Jetcat P70b/5 -> Fuel Pump Voltage  (V)/1
  Jetcat P70b/4 -> Fuel Flow (lbs/min)/1
  Jetcat P70b/3 -> h (slg-ft^2/s)/1
  Jetcat P70b/2 -> RPM/1
  Jetcat P70b/1 -> Thrust (lbf)/1
  tratio/1 -> Jetcat P70b/3
  pratio/1 -> Jetcat P70b/2
  Throttle/1 -> Jetcat P70b/1

== system models/gtm-aero (for V0905)/aero surf ganging/Actuator_GTM_T2 (modified) ==
  cmds : Inport  OutDataType=sfix(16)  OutScaling=2^0
  cmd_stab : Inport  Port=2  OutDataType=sfix(16)  OutScaling=2^0
  Brake : Saturate  UpperLimit=1.0  LowerLimit=0.0
  Bus Selector2 : BusSelector  OutputSignals=ELLOBC,ELLIBC,ELROBC,ELRIBC,AILLC,AILRC,RUDUPC,RUDLOC,SPLLIBC,SPLLOBC,SPLRIBC,SPLROBC,FLAPLIC,FLAPLOC,FLAPRIC,FLAPROC,GEARC,BRAKEC,THROTLC,THROTRC,STEERC
  Gear : Saturate  UpperLimit=1.0  LowerLimit=0.0
  Gear1 : Constant  Value=bias.stabilizer*0  OutDataType=sfix(16)  OutScaling=2^0
  Ground : Ground
  Label : Subsystem
  Mux : Mux  Inputs=22
  Sum : Sum  Inputs=++|  OutDataType=sfix(16)  OutScaling=2^0
  Sum3 : Sum  Inputs=|++  OutDataType=sfix(16)  OutScaling=2^0
  Surface Allocation : Subsystem
  Surface Pos : Outport  OutDataType=sfix(16)  OutScaling=2^0
  wires:
  Sum3/1 -> Mux/17
  Gear1/1 -> Sum3/2
  cmd_stab/1 -> Sum3/1
  Bus Selector2/21 -> Mux/22  "<STEERC>"
  Bus Selector2/20 -> Mux/21  "<THROTRC>"
  Bus Selector2/19 -> Mux/20  "<THROTLC>"
  Surface Allocation/1(O) -> Sum/1
  cmds/1 -> Bus Selector2/1
  Brake/1 -> Mux/19
  Gear/1 -> Mux/18
  Bus Selector2/12 -> Mux/12  "<SPLROBC>"
  Bus Selector2/11 -> Mux/11  "<SPLRIBC>"
  Bus Selector2/10 -> Mux/10  "<SPLLOBC>"
  Bus Selector2/9 -> Mux/9  "<SPLLIBC>"
  Bus Selector2/8 -> Mux/8  "<RUDLOC>"
  Bus Selector2/7 -> Mux/7  "<RUDUPC>"
  Bus Selector2/6 -> Mux/6  "<AILRC>"
  Bus Selector2/5 -> Mux/5  "<AILLC>"
  Bus Selector2/4 -> Mux/4  "<ELRIBC>"
  Bus Selector2/3 -> Mux/3  "<ELROBC>"
  Bus Selector2/2 -> Mux/2  "<ELLIBC>"
  Bus Selector2/1 -> Mux/1  "<ELLOBC>"
  Mux/1 -> Sum/2
  Bus Selector2/18 -> Brake/1  "<BRAKEC>"
  Bus Selector2/17 -> Gear/1  "<GEARC>"
  Bus Selector2/16 -> Mux/16  "<FLAPROC>"
  Bus Selector2/15 -> Mux/15  "<FLAPRIC>"
  Bus Selector2/14 -> Mux/14  "<FLAPLOC>"
  Bus Selector2/13 -> Mux/13  "<FLAPLIC>"
  Ground/1 -> Surface Allocation/1(I)
  Label/1(O) -> Surface Pos/1
  Sum/1 -> Label/1(I)

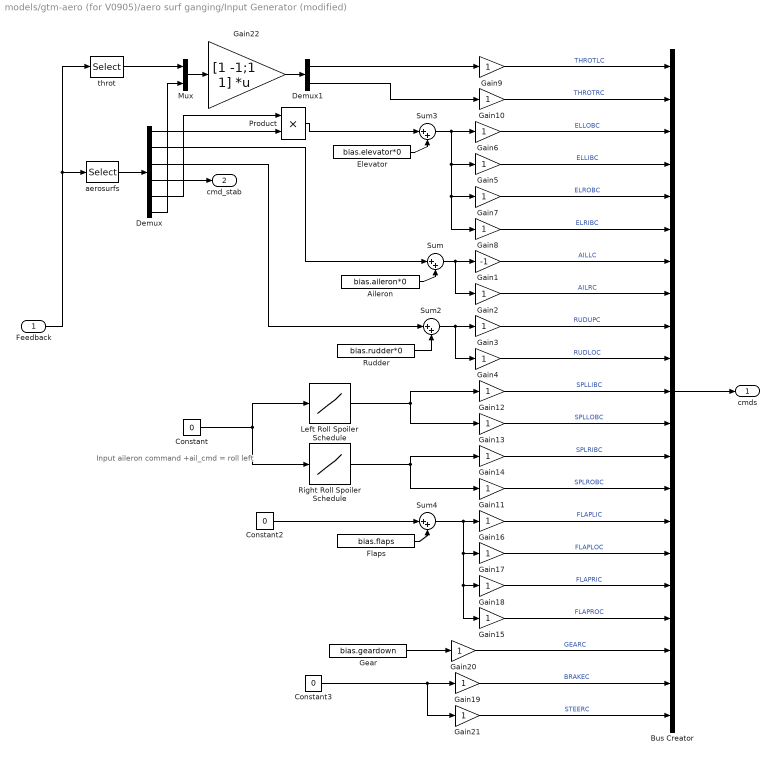
== system models/gtm-aero (for V0905)/aero surf ganging/Input Generator (modified) ==
  note: Input aileron command
      | +ail_cmd = roll left
  Feedback : Inport  OutDataType=sfix(16)  OutScaling=2^0
  Aileron : Constant  Value=bias.aileron*0  OutDataType=sfix(16)  OutScaling=2^0
  Bus Creator : BusCreator  Inputs=21
  Constant : Constant  Value=0  OutDataType=sfix(16)  OutScaling=2^0
  Constant2 : Constant  Value=0  OutDataType=sfix(16)  OutScaling=2^0
  Constant3 : Constant  Value=0  OutDataType=sfix(16)  OutScaling=2^0
  Demux : Demux  Outputs=6
  Demux1 : Demux  Outputs=2
  Elevator : Constant  Value=bias.elevator*0  OutDataType=sfix(16)  OutScaling=2^0
  Flaps : Constant  Value=bias.flaps  OutDataType=sfix(16)  OutScaling=2^0
  Gain1 : Gain  Gain=-1  ParameterDataType=sfix(16)  ParameterScaling=2^0  OutDataType=sfix(16)  OutScaling=2^0  SaturateOnIntegerOverflow=on  OutDataTypeStr=Inherit: Same as input  ParamDataTypeStr=Inherit: Same as input
  Gain{2..21} (20 alike) : Gain  ParameterDataType=sfix(16)  ParameterScaling=2^0  OutDataType=sfix(16)  OutScaling=2^0  SaturateOnIntegerOverflow=on  OutDataTypeStr=Inherit: Same as input  ParamDataTypeStr=Inherit: Same as input
  Gain22 : Gain  Gain=[1 -1;1 1]  Multiplication=Matrix(K*u)  ParameterDataType=sfix(16)  ParameterScaling=2^0  OutDataType=sfix(16)  OutScaling=2^0  SaturateOnIntegerOverflow=on  OutDataTypeStr=Inherit: Same as input  ParamDataTypeStr=Inherit: Same as input
  Gear : Constant  Value=bias.geardown  OutDataType=sfix(16)  OutScaling=2^0
  Left Roll Spoiler Schedule : Lookup  InputValues="[-20\t-11.76\t-2.36\t0\t2.36\t11.76\t20\t]"  Table=[0 0 0 0 0 9 45]  LookUpMeth=Interpolation-Use End Values  OutDataType=sfix(16)  OutScaling=2^0
  Mux : Mux  Inputs=2
  Product : Product  OutDataType=sfix(16)  OutScaling=2^0  RndMeth=Zero
  Right Roll Spoiler Schedule : Lookup  InputValues="[-20\t-11.76\t-2.36\t0\t2.36\t11.76\t20\t]"  Table=[45 9 0 0 0 0 0]  LookUpMeth=Interpolation-Use End Values  OutDataType=sfix(16)  OutScaling=2^0
  Rudder : Constant  Value=bias.rudder*0  OutDataType=sfix(16)  OutScaling=2^0
  Sum{,2..4} (4 alike) : Sum  Inputs=|++  OutDataType=sfix(16)  OutScaling=2^0
  aerosurfs : Selector  InputPortWidth=num_u  IndexOptions=Index vector (dialog)  Indices=vane_idx  OutputSizes=1
  throt : Selector  InputPortWidth=num_u  IndexOptions=Index vector (dialog)  Indices=throttle_idx  OutputSizes=1
  cmds : Outport  OutDataType=sfix(16)  OutScaling=2^0
  cmd_stab : Outport  Port=2  OutDataType=sfix(16)  OutScaling=2^0
  wires:
  Demux1/2 -> Gain10/1
  Demux1/1 -> Gain9/1
  Gain22/1 -> Demux1/1
  Mux/1 -> Gain22/1
  throt/1 -> Mux/1
  Demux/6 -> Mux/2
  Demux/5 -> Product/1
  Demux/1 -> Product/2
  Product/1 -> Sum3/1
  Demux/4 -> cmd_stab/1
  aerosurfs/1 -> Demux/1
  Gain21/1 -> Bus Creator/21  "STEERC"
  Gain20/1 -> Bus Creator/19  "GEARC"
  Feedback/1 -> aerosurfs/1, throt/1
  Bus Creator/1 -> cmds/1
  Constant3/1 -> Gain21/1, Gain19/1
  Gear/1 -> Gain20/1
  Gain19/1 -> Bus Creator/20  "BRAKEC"
  Demux/3 -> Sum2/1
  Demux/2 -> Sum/1
  Sum4/1 -> Gain15/1, Gain18/1, Gain17/1, Gain16/1
  Constant2/1 -> Sum4/1
  Flaps/1 -> Sum4/2
  Rudder/1 -> Sum2/2
  Sum2/1 -> Gain4/1, Gain3/1
  Sum/1 -> Gain2/1, Gain1/1
  Elevator/1 -> Sum3/2
  Aileron/1 -> Sum/2
  Sum3/1 -> Gain8/1, Gain7/1, Gain5/1, Gain6/1
  Gain4/1 -> Bus Creator/10  "RUDLOC"
  Gain3/1 -> Bus Creator/9  "RUDUPC"
  Gain2/1 -> Bus Creator/8  "AILRC"
  Gain1/1 -> Bus Creator/7  "AILLC"
  Gain8/1 -> Bus Creator/6  "ELRIBC"
  Gain7/1 -> Bus Creator/5  "ELROBC"
  Gain6/1 -> Bus Creator/3  "ELLOBC"
  Gain5/1 -> Bus Creator/4  "ELLIBC"
  Gain10/1 -> Bus Creator/2  "THROTRC"
  Gain9/1 -> Bus Creator/1  "THROTLC"
  Gain15/1 -> Bus Creator/18  "FLAPROC"
  Gain18/1 -> Bus Creator/17  "FLAPRIC"
  Gain17/1 -> Bus Creator/16  "FLAPLOC"
  Gain16/1 -> Bus Creator/15  "FLAPLIC"
  Gain11/1 -> Bus Creator/14  "SPLROBC"
  Gain14/1 -> Bus Creator/13  "SPLRIBC"
  Gain13/1 -> Bus Creator/12  "SPLLOBC"
  Gain12/1 -> Bus Creator/11  "SPLLIBC"
  Left Roll Spoiler Schedule/1 -> Gain12/1, Gain13/1
  Right Roll Spoiler Schedule/1 -> Gain14/1, Gain11/1
  Constant/1 -> Left Roll Spoiler Schedule/1, Right Roll Spoiler Schedule/1

== system models/gtm-aero/A/C parameters/Inertia/Mass/CG Shift/DamageEffects ==
  In : Inport  OutDataType=sfix(16)  OutScaling=2^0
  Gain1 : Constant  Value=dInertiaDamage  OutDataType=sfix(16)  OutScaling=2^0
  Squeeze2 : Squeeze
  Value(ndx,:) : Selector  NumberOfDimensions=2  IndexMode=Zero-based  InputPortWidth=3  IndexOptions=Index vector (port),Select all  Indices=[1 3],1  OutputSizes=1,1
  dInertia : Outport  OutDataType=sfix(16)  OutScaling=2^0
  wires:
  Squeeze2/1 -> dInertia/1
  Value(ndx,:)/1 -> Squeeze2/1
  Gain1/1 -> Value(ndx,:)/1
  In/1 -> Value(ndx,:)/2

== system models/gtm-aero/A/C parameters/Inertia/Mass/CG Shift/FuelBurnEffects ==
  In : Inport  OutDataType=sfix(16)  OutScaling=2^0
  Mux : Mux
  Polyval : Polyval_lib/Polyval  SystemSampleTime=-1  p=Ixx_model
  Polyval1 : Polyval_lib/Polyval  SystemSampleTime=-1  p=Iyy_model
  Polyval2 : Polyval_lib/Polyval  SystemSampleTime=-1  p=Izz_model
  xCG6 : Constant  Value=zeros(1,3)  OutDataType=sfix(16)  OutScaling=2^0
  dInertia : Outport  OutDataType=sfix(16)  OutScaling=2^0
  wires:
  Mux/1 -> dInertia/1
  Polyval2/1 -> Mux/3
  Polyval1/1 -> Mux/2
  Polyval/1 -> Mux/1
  xCG6/1 -> Mux/4
  In/1 -> Polyval2/1, Polyval1/1, Polyval/1

== system models/gtm-aero/A/C parameters/Inertia/Mass/CG Shift/cg/weight ==
  DamageCase : Inport  OutDataType=sfix(16)  OutScaling=2^0
  Gain1 : Constant  Value=dMassDamage  OutDataType=sfix(16)  OutScaling=2^0
  Gain2 : Constant  Value=dCGDamage  OutDataType=sfix(16)  OutScaling=2^0
  Squeeze1 : Squeeze
  Squeeze2 : Squeeze
  Value(ndx,:) : Selector  IndexMode=Zero-based  IndexOptions=Index vector (port)  Indices=[1 3]  OutputSizes=1
  Value(ndx,:)1 : Selector  NumberOfDimensions=2  IndexMode=Zero-based  InputPortWidth=3  IndexOptions=Index vector (port),Select all  Indices=[1 3],1  OutputSizes=1,1
  dCG : Outport  OutDataType=sfix(16)  OutScaling=2^0
  dweight : Outport  Port=2  OutDataType=sfix(16)  OutScaling=2^0
  wires:
  Squeeze2/1 -> dweight/1
  Squeeze1/1 -> dCG/1
  Value(ndx,:)/1 -> Squeeze2/1
  Gain1/1 -> Value(ndx,:)/1
  DamageCase/1 -> Value(ndx,:)1/2, Value(ndx,:)/2
  Value(ndx,:)1/1 -> Squeeze1/1
  Gain2/1 -> Value(ndx,:)1/1

== system models/gtm-aero/Aero_GTM_T2/Coefficent Evaluation/3D Vector Cross Product ==
  A : Inport  OutDataType=sfix(16)  OutScaling=2^0
  B : Inport  Port=2  OutDataType=sfix(16)  OutScaling=2^0
  Demux : Demux  Outputs=3
  Demux1 : Demux  Outputs=3
  Gain : Gain  Gain=-1  ParameterDataType=sfix(16)  ParameterScaling=2^0  OutDataType=sfix(16)  OutScaling=2^0  SaturateOnIntegerOverflow=on  OutDataTypeStr=Inherit: Same as input  ParamDataTypeStr=Inherit: Same as input
  Ground : Ground
  Mux : Mux  Inputs=9
  Product : Product  Multiplication=Matrix(*)  OutDataType=sfix(16)  OutScaling=2^0  SaturateOnIntegerOverflow=on  OutDataTypeStr=Inherit: Same as first input
  Reshape : Reshape  OutputDimensionality=Customize  OutputDimensions=[3,3]
  Reshape1 : Reshape  OutputDimensions=[3,3]
  AxB : Outport  OutDataType=sfix(16)  OutScaling=2^0
  wires:
  B/1 -> Reshape1/1
  Reshape/1 -> Product/1
  Mux/1 -> Reshape/1
  Demux1/1 -> Mux/8
  Demux/2 -> Mux/7
  Demux/1 -> Mux/6
  Demux1/3 -> Mux/4
  Demux1/2 -> Mux/3
  Demux/3 -> Mux/2
  Gain/1 -> Demux1/1
  Ground/1 -> Mux/9, Mux/5, Mux/1
  Product/1 -> AxB/1
  A/1 -> Gain/1, Demux/1
  Reshape1/1 -> Product/2

== system models/gtm-aero/Aero_GTM_T2/Dynamic Derviatives/Forced Oscillation with Damage Increments ==
  alpha : Inport  OutDataType=sfix(16)  OutScaling=2^0
  TAS : Inport  Port=2  OutDataType=sfix(16)  OutScaling=2^0
  pqr : Inport  Port=3  OutDataType=sfix(16)  OutScaling=2^0
  AC_Params : Inport  Port=4  OutDataType=sfix(16)  OutScaling=2^0
  DamageCase : Inport  Port=5  OutDataType=sfix(16)  OutScaling=2^0
  Action Port : ActionPort
  Add : Sum  Inputs=+++  OutDataType=sfix(16)  OutScaling=2^-10
  Add1 : Sum  OutDataType=sfix(16)  OutScaling=2^-10
  Assignment to  CY : Assignment  IndexMode=Zero-based  IndexOptions=Index vector (dialog)  Indices=1  OutputSizes=[1 1]
  Constant4 : Constant  Value=zeros(6,1)  OutDataType=sfix(16)  OutScaling=2^0
  Damage Effects-Increments : Subsystem
  Damage Effects-Scaling : Subsystem
  Forced Oscillation : Subsystem
  Normalize : Subsystem
  Product1 : Product  OutDataType=sfix(16)  OutScaling=2^0  RndMeth=Zero
  Product2 : Product  OutDataType=sfix(16)  OutScaling=2^0  RndMeth=Zero
  Product3 : Product  OutDataType=sfix(16)  OutScaling=2^0  RndMeth=Zero
  dC6 : Outport  OutDataType=sfix(16)  OutScaling=2^0
  wires:
  Assignment to  CY/1 -> Add1/1
  Add/1 -> Add1/2
  Product2/1 -> Add/1
  Product1/1 -> Add/2
  Product3/1 -> Add/3
  Forced Oscillation/3(dC6_r) -> Product3/2
  Forced Oscillation/2(dC6_q) -> Product1/2
  Forced Oscillation/1(dC6_p) -> Product2/2
  Normalize/1(pqrhat) -> Damage Effects-Increments/2(pqr), Forced Oscillation/2(pqr)
  AC_Params/1 -> Normalize/3(AC_Params)
  TAS/1 -> Normalize/2(TAS)
  pqr/1 -> Normalize/1(pqr)
  Add1/1 -> dC6/1
  Constant4/1 -> Assignment to  CY/1
  Damage Effects-Increments/1(Increment) -> Assignment to  CY/2
  Damage Effects-Scaling/3(Scaling_p) -> Product2/1
  Damage Effects-Scaling/2(Scaling_q) -> Product1/1
  Damage Effects-Scaling/1(Scaling_r) -> Product3/1
  DamageCase/1 -> Damage Effects-Increments/3(DamageCase), Damage Effects-Scaling/2(DamageCase)
  alpha/1 -> Damage Effects-Increments/1(alpha), Damage Effects-Scaling/1(alpha), Forced Oscillation/1(alpha)

== system models/gtm-aero/Aero_GTM_T2/Dynamic Derviatives/Rotary Blended  UnDamaged Case ==
  alpha : Inport  OutDataType=sfix(16)  OutScaling=2^0
  beta : Inport  Port=2  OutDataType=sfix(16)  OutScaling=2^0
  TAS : Inport  Port=3  OutDataType=sfix(16)  OutScaling=2^0
  pqr : Inport  Port=4  OutDataType=sfix(16)  OutScaling=2^0
  AC_Params : Inport  Port=5  OutDataType=sfix(16)  OutScaling=2^0
  Action Port : ActionPort
  Add : Sum  Inputs=++++  OutDataType=sfix(16)  OutScaling=2^-10
  Blending Function : Stateflow chart
  Bus Selector2 : BusSelector  OutputSignals=B,Cbar
  Forced Oscillation : Subsystem
  Rotary Balance : Subsystem
  Saturation : Saturate
  Saturation1 : Saturate  UpperLimit=10000  LowerLimit=1
  Signal Specification : SignalSpecification  Dimensions=3  OutDataType=sfix(16)  OutScaling=2^0
  dC6 : Outport  OutDataType=sfix(16)  OutScaling=2^0
  wires:
  Forced Oscillation/3(dC6_r) -> Add/4
  Forced Oscillation/2(dC6_q) -> Add/3
  Forced Oscillation/1(dC6_p) -> Add/2
  Rotary Balance/1(dC6) -> Add/1
  Add/1 -> dC6/1
  Bus Selector2/2 -> Blending Function/6(Cbar)  "<Cbar>"
  pqr/1 -> Signal Specification/1
  Saturation1/1 -> Blending Function/3(tas)
  Saturation/1 -> Rotary Balance/3(w)
  [alpha] -> Forced Oscillation/1(alpha)
  [beta] -> Rotary Balance/2(beta)
  [alpha] -> Rotary Balance/1(alpha)
  [beta] -> Blending Function/2(beta)
  beta/1 -> [beta]
  alpha/1 -> [alpha]
  [alpha] -> Blending Function/1(alpha)
  AC_Params/1 -> Bus Selector2/1
  TAS/1 -> Saturation1/1
  Bus Selector2/1 -> Blending Function/5(B)  "<B>"
  Blending Function/2(pqr_osc) -> Forced Oscillation/2(pqr)
  Blending Function/1(omega) -> Saturation/1
  Signal Specification/1 -> Blending Function/4(pqr)

== system models/gtm-aero/aero surf ganging/Actuator_GTM_T2 (modified)/Label ==
  I : Inport  OutDataType=sfix(16)  OutScaling=2^0
  Bus Creator : BusCreator  Inputs=22
  Demux : Demux  Outputs=22
  O : Outport  OutDataType=sfix(16)  OutScaling=2^0
  wires:
  I/1 -> Demux/1
  Bus Creator/1 -> O/1
  Demux/2 -> Bus Creator/2  "ELLIB"
  Demux/3 -> Bus Creator/3  "ELROB"
  Demux/4 -> Bus Creator/4  "ELRIB"
  Demux/5 -> Bus Creator/5  "AILL"
  Demux/6 -> Bus Creator/6  "AILR"
  Demux/7 -> Bus Creator/7  "RUDU"
  Demux/8 -> Bus Creator/8  "RUDL"
  Demux/9 -> Bus Creator/9  "SPLLIB"
  Demux/10 -> Bus Creator/10  "SPLLOB"
  Demux/11 -> Bus Creator/11  "SPLRIB"
  Demux/12 -> Bus Creator/12  "SPLROB"
  Demux/13 -> Bus Creator/13  "FLAPLIB"
  Demux/14 -> Bus Creator/14  "FLAPLOB"
  Demux/15 -> Bus Creator/15  "FLAPRIB"
  Demux/16 -> Bus Creator/16  "FLAPROB"
  Demux/17 -> Bus Creator/17  "STAB"
  Demux/18 -> Bus Creator/18  "GEAR"
  Demux/1 -> Bus Creator/1  "ELLOB"
  Demux/19 -> Bus Creator/19  "BRAKE"
  Demux/20 -> Bus Creator/20  "THROTL"
  Demux/21 -> Bus Creator/21  "THROTR"
  Demux/22 -> Bus Creator/22  "STEER"
